simulink model "chap8_10sim"  (R2015a)
settings: Solver=ode45  StartTime=0.0  StopTime=100  RelTol=1e-3
settings Model: Creator=zhr  LastModifiedBy=zhr

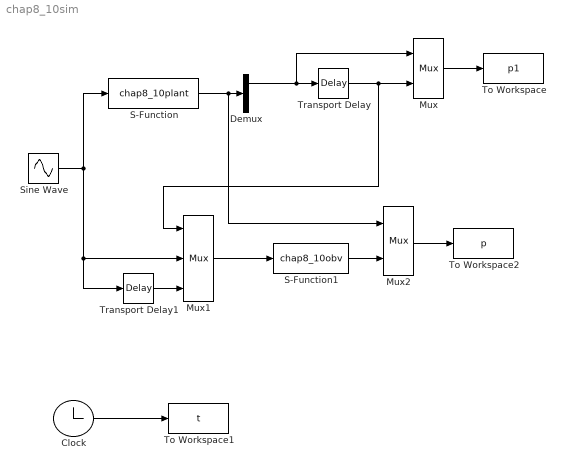
== system chap8_10sim ==
  Clock : Clock
  Demux : Demux  Outputs=2
  Mux : Mux  Inputs=2
  Mux1 : Mux  Inputs=3
  Mux2 : Mux  Inputs=2
  S-Function : S-Function  FunctionName=chap8_10plant
  S-Function1 : S-Function  FunctionName=chap8_10obv
  Sine Wave : Sin  SampleTime=0
  To Workspace : ToWorkspace  VariableName=p1  SampleTime=-1
  To Workspace1 : ToWorkspace  VariableName=t  SampleTime=-1
  To Workspace2 : ToWorkspace  VariableName=p  SampleTime=-1
  Transport Delay : TransportDelay
  Transport Delay1 : TransportDelay
  wires:
  Clock/1 -> To Workspace1/1
  S-Function/1 -> Mux2/1, Demux/1
  Demux/1 -> Mux/1, Transport Delay/1
  Transport Delay/1 -> Mux1/1, Mux/2
  Mux/1 -> To Workspace/1
  Sine Wave/1 -> S-Function/1, Transport Delay1/1, Mux1/2
  Transport Delay1/1 -> Mux1/3
  Mux1/1 -> S-Function1/1
  S-Function1/1 -> Mux2/2
  Mux2/1 -> To Workspace2/1
